simulink model "RocketLanderSimulation_testing"  (R2022b)
settings: Solver=VariableStepAuto  StartTime=0.0  StopTime=15  RelTol=1e-3
undefined symbols (not defined in the file or in its folder): pLander, references, u0, x0
libraries: simulink x1, mpclib x1
settings Model: Creator=The MathWorks, Inc.  LastModifiedBy=The MathWorks, Inc.
settings DebuggingCC: UnconnectedInputMsg=warning  UnconnectedOutputMsg=warning  UnconnectedLineMsg=warning
settings ModelReferenceCC: EnableRefExpFcnMdlSchedulingChecks=on
settings RTWCC: DLArmComputeVersion=19.05

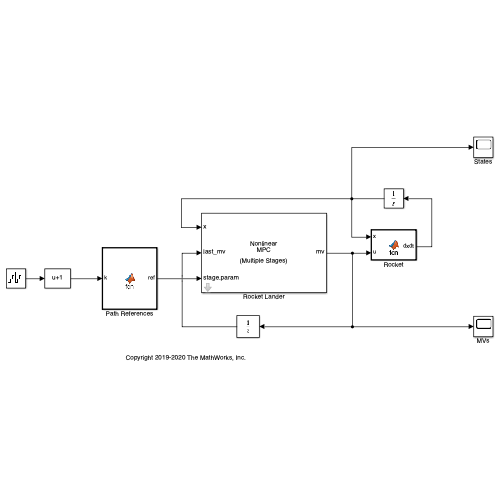
[thumbnail: Simulink's stored preview of the top-level diagram]
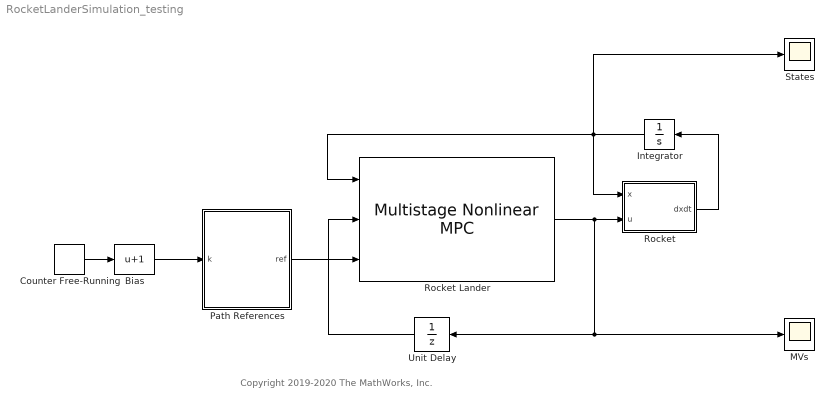
== system RocketLanderSimulation_testing ==
  note: Copyright 2019-2020 The MathWorks, Inc.
  Bias : Bias  Bias=1  SaturateOnIntegerOverflow=off
  Counter Free-Running : simulink/Sources/Counter Free-Running  NumBits=16  tsamp=Ts
  Integrator : Integrator  InitialCondition=x0
  MVs : Scope
  Path References : MATLAB Function  TreatAsAtomicUnit=on
  Rocket : MATLAB Function  TreatAsAtomicUnit=on
  Rocket Lander : mpclib/Multistage Nonlinear MPC  SCDEnableBlockLinearizationSpecification=on  nlmpcobj=lander  UseObjectTs=on  UseMEX=off  md_enabled=off  stateparam_enabled=off  stageparam_enabled=on  cost_enabled=off  mvseq_enabled=off  stateseq_enabled=off  slack_enabled=off  status_enabled=off  mv_min=off  mv_max=off  mvrate_min=off  mvrate_max=off  state_min=off  state_max=off  terminal_state=off  nlp_initialize=off
  States : Scope
  Unit Delay : UnitDelay  InitialCondition=u0  SampleTime=-1  HasFrameUpgradeWarning=on
  wires:
  Rocket Lander/1 -> Unit Delay/1, MVs/1, Rocket/2(u)
  Rocket/1(dxdt) -> Integrator/1
  Integrator/1 -> States/1, Rocket Lander/1, Rocket/1(x)
  Unit Delay/1 -> Rocket Lander/2
  Path References/1(ref) -> Rocket Lander/3
  Counter Free-Running/1 -> Bias/1
  Bias/1 -> Path References/1(k)

== matlab function RocketLanderSimulation_testing/Rocket ==
  data: x input; u input; dxdt output
function dxdt = fcn(x,u)
dxdt = RocketStateFcn(x,u);

== matlab function RocketLanderSimulation_testing/Path References ==
  data: k input; ref output; references parameter; pLander parameter
function ref = fcn(k,references,pLander)
ref = RocketLanderReferenceSignal(k,references,pLander);
